simulink library "CRYP_PF_MASTER"  (Simulink 8.5)
settings: Solver=ode45  StartTime=0.0  StopTime=10.0  RelTol=1e-3
libraries: cdsEpicsOut x53, cdsFilt x16, cdsTP x16, VIS_LIB x8, cdsFunctionCall x5, cdsFiltCtrl x4, cdsMuxMatrix x4, cdsEpicsIn x2, lockin x2, QPD x2, cdsRms x2, FOUROSEM_COILOUTF_MASTER x1
(part 1 of 3)
settings Model: Creator=controls  LastModifiedBy=controls

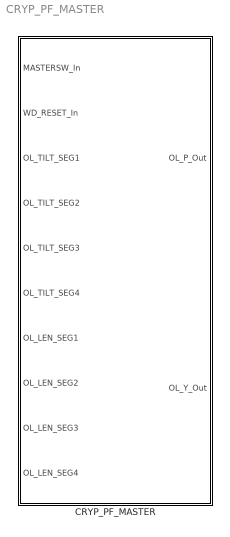
== system CRYP_PF_MASTER ==
  CRYP_PF_MASTER : Subsystem

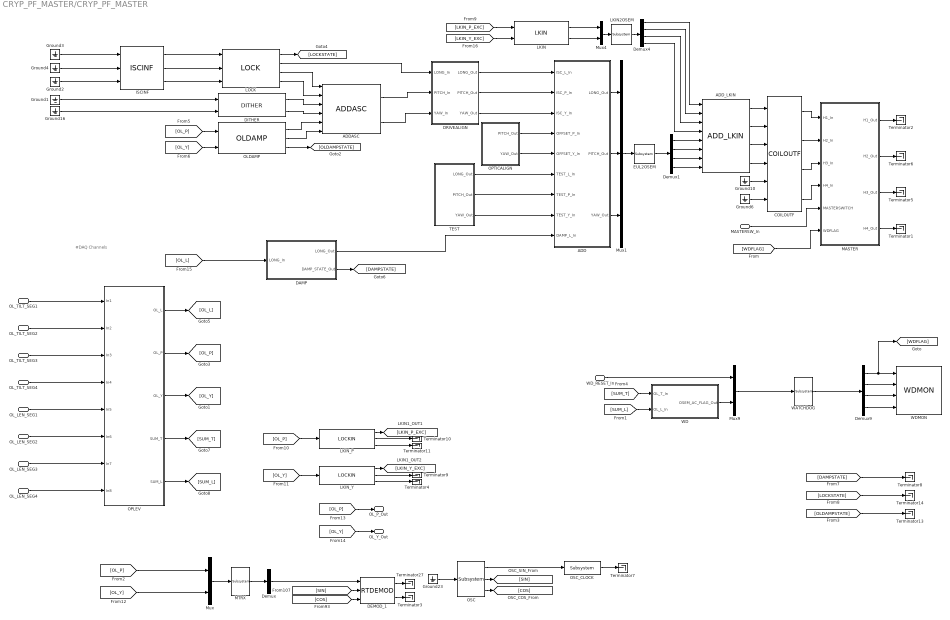
== system CRYP_PF_MASTER/CRYP_PF_MASTER ==
  note: #DAQ Channels
  MASTERSW_In : Inport
  WD_RESET_In : Inport  Port=2
  OL_TILT_SEG1 : Inport  Port=3
  OL_TILT_SEG2 : Inport  Port=4
  OL_TILT_SEG3 : Inport  Port=5
  OL_TILT_SEG4 : Inport  Port=6
  OL_LEN_SEG1 : Inport  Port=7
  OL_LEN_SEG2 : Inport  Port=8
  OL_LEN_SEG3 : Inport  Port=9
  OL_LEN_SEG4 : Inport  Port=10
  ADD : Subsystem
  ADDASC : VIS_LIB/ADDASC
  ADD_LKIN : VIS_LIB/ADD_LKIN
  COILOUTF : FOUROSEM_COILOUTF_MASTER/COILOUTF
  DAMP : Subsystem
  DEMOD_1 : rtdemod/RTDEMOD  Tag=top_names
  DITHER : VIS_LIB/DITHER
  DRIVEALIGN : Subsystem
  Demux : Demux  Outputs=1
  Demux1 : Demux
  Demux4 : Demux
  Demux9 : Demux
  EUL2OSEM : cdsMuxMatrix/Subsystem  Tag=cdsMuxMatrix  Description=Any size matrix. Inputs and outputs must be connected using Mux and Demux parts.
      settings: AttributesFormatString=%<Tag>
  Ground{1..4,6,10,16,23} (8 alike) : Ground
  ISCINF : VIS_LIB/ISCINF
  LKIN : VIS_LIB/LKIN
  LKIN2OSEM : cdsMuxMatrix/Subsystem  Tag=cdsMuxMatrix  Description=Any size matrix. Inputs and outputs must be connected using Mux and Demux parts.
      settings: AttributesFormatString=%<Tag>
  LKIN_P : lockin/LOCKIN  Description=ADL=LOCKIN.adl
      settings: AttributesFormatString=%<Tag>
  LKIN_Y : lockin/LOCKIN  Description=ADL=LOCKIN.adl
      settings: AttributesFormatString=%<Tag>
  LOCK : VIS_LIB/LOCK
  MASTER : Subsystem  AncestorBlock=VIS_LIB/MASTER
  MTRX : cdsMuxMatrix/Subsystem  Tag=cdsMuxMatrix  Description=Any size matrix. Inputs and outputs must be connected using Mux and Demux parts.
      settings: AttributesFormatString=%<Tag>
  Mux : Mux  Inputs=2
  Mux1 : Mux  Inputs=3
  Mux4 : Mux  Inputs=2
  Mux9 : Mux  Inputs=2
  OLDAMP : VIS_LIB/OLDAMP
  OPLEV : Subsystem
  OPTICALIGN : Subsystem
  OSC : cdsOsc/Subsystem  Tag=cdsOsc  Description=Oscillator
      settings: AttributesFormatString=%<Tag>
  OSC_CLOCK : cdsEpicsOut/Subsystem  Tag=cdsEpicsOutput  Description=|
      | Purpose:                                          
      | Output a FE signal to an EPICS channel.           
      |                                                   
      | Operation:                                        
      | Takes input value and passes it to EPICS record.  
      |                                                   
      | Usage:                                            
      | Name the part with the desired EPICS rrecord name.
      settings: AttributesFormatString=%<Tag>
  TEST : Subsystem
  Terminator{1..11,13..14,27} (14 alike) : Terminator
  WATCHDOG : cdsFunctionCall/Subsystem  Tag=cdsFunctionCall  Description=inline OSEMWATCHDOG /opt/rtcds/userapps/release/vis/common/src/WATCHDOG.c
      settings: AttributesFormatString=%<Tag>\n%<Description>
  WD : Subsystem
  WDMON : VIS_LIB/WDMON
  OL_P_Out : Outport
  OL_Y_Out : Outport  Port=2
  wires:
  [SUM_L] -> WD/2(OL_L_In)
  [SUM_T] -> WD/1(OL_T_In)
  DAMP/1(LONG_Out) -> ADD/9(DAMP_L_In)
  DAMP/2(DAMP_STATE_Out) -> [DAMPSTATE]
  [OL_L] -> DAMP/1(LONG_In)
  OPTICALIGN/2(YAW_Out) -> ADD/5(OFFSET_Y_In)
  OPTICALIGN/1(PITCH_Out) -> ADD/4(OFFSET_P_In)
  LOCK/3 -> ADDASC/1
  TEST/3(YAW_Out) -> ADD/8(TEST_Y_In)
  TEST/2(PITCH_Out) -> ADD/7(TEST_P_In)
  TEST/1(LONG_Out) -> ADD/6(TEST_L_In)
  Ground10/1 -> COILOUTF/5
  Ground6/1 -> COILOUTF/6
  WD_RESET_In/1 -> Mux9/1
  COILOUTF/4 -> MASTER/4(H4_In)
  COILOUTF/3 -> MASTER/3(H3_In)
  COILOUTF/2 -> MASTER/2(H2_In)
  COILOUTF/1 -> MASTER/1(H1_In)
  [WDFLAG] -> MASTER/6(WDFLAG)
  Mux9/1 -> WATCHDOG/1
  WATCHDOG/1 -> Demux9/1
  Demux9/4 -> WDMON/4
  Demux9/3 -> WDMON/3
  Demux9/2 -> WDMON/2
  Demux9/1 -> WDMON/1, [WDFLAG]
  EUL2OSEM/1 -> Demux1/1
  Mux1/1 -> EUL2OSEM/1
  Ground1/1 -> DITHER/1
  Ground16/1 -> DITHER/2
  [OL_P] -> OLDAMP/1
  [OL_Y] -> OLDAMP/2
  LOCK/4 -> ADDASC/2
  DITHER/1 -> ADDASC/3
  DITHER/2 -> ADDASC/4
  OLDAMP/1 -> ADDASC/5
  OLDAMP/2 -> ADDASC/6
  ADD/3(YAW_Out) -> Mux1/3
  ADD/2(PITCH_Out) -> Mux1/2
  ADD/1(LONG_Out) -> Mux1/1
  LOCK/2 -> DRIVEALIGN/1(LONG_In)
  ADDASC/1 -> DRIVEALIGN/2(PITCH_In)
  ADDASC/2 -> DRIVEALIGN/3(YAW_In)
  DRIVEALIGN/1(LONG_Out) -> ADD/1(ISC_L_In)
  DRIVEALIGN/2(PITCH_Out) -> ADD/2(ISC_P_In)
  DRIVEALIGN/3(YAW_Out) -> ADD/3(ISC_Y_In)
  OLDAMP/3 -> [OLDAMPSTATE]
  MASTER/1(H1_Out) -> Terminator2/1
  MASTER/2(H2_Out) -> Terminator6/1
  MASTER/3(H3_Out) -> Terminator5/1
  MASTER/4(H4_Out) -> Terminator1/1
  Mux4/1 -> LKIN2OSEM/1
  LKIN2OSEM/1 -> Demux4/1
  Demux4/1 -> ADD_LKIN/1
  LKIN/1 -> Mux4/1
  LKIN/2 -> Mux4/2
  Demux4/2 -> ADD_LKIN/2
  Demux4/3 -> ADD_LKIN/3
  Demux4/4 -> ADD_LKIN/4
  Demux1/1 -> ADD_LKIN/5
  Demux1/2 -> ADD_LKIN/6
  Demux1/3 -> ADD_LKIN/7
  Demux1/4 -> ADD_LKIN/8
  ADD_LKIN/1 -> COILOUTF/1
  ADD_LKIN/2 -> COILOUTF/2
  ADD_LKIN/3 -> COILOUTF/3
  ADD_LKIN/4 -> COILOUTF/4
  MASTERSW_In/1 -> MASTER/5(MASTERSWITCH)
  [DAMPSTATE] -> Terminator8/1
  [LOCKSTATE] -> Terminator14/1
  [OLDAMPSTATE] -> Terminator13/1
  LOCK/1 -> [LOCKSTATE]
  [LKIN_P_EXC] -> LKIN/1
  [LKIN_Y_EXC] -> LKIN/2
  WD/1(OSEM_AC_FLAG_Out) -> Mux9/2
  Ground2/1 -> ISCINF/3
  Ground3/1 -> ISCINF/1
  Ground4/1 -> ISCINF/2
  ISCINF/1 -> LOCK/1
  ISCINF/2 -> LOCK/2
  ISCINF/3 -> LOCK/3
  Mux/1 -> MTRX/1
  MTRX/1 -> Demux/1
  Demux/1 -> DEMOD_1/1
  [SIN] -> DEMOD_1/2
  [COS] -> DEMOD_1/3
  DEMOD_1/1 -> Terminator27/1
  DEMOD_1/2 -> Terminator3/1
  Ground23/1 -> OSC/1
  OSC/1 -> OSC_CLOCK/1
  OSC_CLOCK/1 -> Terminator7/1
  OSC/2 -> [SIN]
  OSC/3 -> [COS]
  [OL_P] -> Mux/1
  [OL_Y] -> Mux/2
  [OL_P] -> LKIN_P/1
  LKIN_P/2 -> Terminator10/1
  LKIN_P/3 -> Terminator11/1
  LKIN_P/1 -> [LKIN_P_EXC]
  LKIN_Y/1 -> [LKIN_Y_EXC]
  [OL_Y] -> LKIN_Y/1
  LKIN_Y/2 -> Terminator9/1
  LKIN_Y/3 -> Terminator4/1
  [OL_P] -> OL_P_Out/1
  [OL_Y] -> OL_Y_Out/1
  OPLEV/5(SUM_L) -> [SUM_L]
  OPLEV/4(SUM_T) -> [SUM_T]
  OPLEV/3(OL_Y) -> [OL_Y]
  OPLEV/2(OL_P) -> [OL_P]
  OPLEV/1(OL_L) -> [OL_L]
  OL_TILT_SEG3/1 -> OPLEV/3(In3)
  OL_LEN_SEG4/1 -> OPLEV/8(In8)
  OL_LEN_SEG3/1 -> OPLEV/7(In7)
  OL_LEN_SEG2/1 -> OPLEV/6(In6)
  OL_LEN_SEG1/1 -> OPLEV/5(In5)
  OL_TILT_SEG4/1 -> OPLEV/4(In4)
  OL_TILT_SEG2/1 -> OPLEV/2(In2)
  OL_TILT_SEG1/1 -> OPLEV/1(In1)

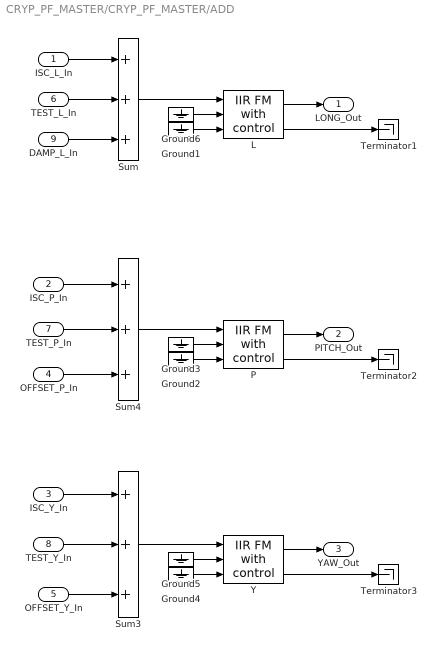
== system CRYP_PF_MASTER/CRYP_PF_MASTER/ADD ==
  ISC_L_In : Inport
  ISC_P_In : Inport  Port=2
  ISC_Y_In : Inport  Port=3
  OFFSET_P_In : Inport  Port=4
  OFFSET_Y_In : Inport  Port=5
  TEST_L_In : Inport  Port=6
  TEST_P_In : Inport  Port=7
  TEST_Y_In : Inport  Port=8
  DAMP_L_In : Inport  Port=9
  Ground{1..6} (6 alike) : Ground
  L : cdsFiltCtrl/IIR FM with control  Tag=cdsFiltCtrl  Description=|
      | cdsFiltCntrl is the standard IIR filter module (exactly the same as cdsFilt) but with added control data output 'Ctrl'. Filter module digital signal output appears on the first output, which is called 'Val'. 'Ctrl' output has a bit pattern encoding the state of filter's on/off switches (FM1 through FM10). The bit values are:
      |                                                                                                                                                                                                                                                                                                                                       
      | module 	hex	dec                                                                                                                                                                                                                                                                                                                       
      | -----------------------                                                                                                                                                                                                                                                                                                               
      | FM1	0x20                    32                                                                                                                                                                                                                                                                                                        
      | FM2	0x80                     128                                                                                                                                                                                                                                                                                                      
      | FM3	0x200                   512                                                                                                                                                                                                                                                                                                       
      | FM4	0x800                   2048                                                                                                                                                                                                                                                                                                      
      | FM5	0x2000                 8192                                                                                                                                                                                                                                                                                                       
      | FM6	0x8000                 32768                                                                                                                                                                                                                                                                                                      
      | FM7	0x20000                131072                                                                                                                                                                                                                                                                                                     
      | FM8	0x80000                 524288                                                                                                                                                                                                                                                                                                    
      | FM9	0x200000               2097152                                                                                                                                                                                                                                                                                                    
      | FM10	0x800000               8388608                                                                                                                                                                                                                                                                                                   
      |                                                                                                                                                                                                                                                                                                                                       
      | This bit data can be used to drive some other switches or it can be output using a binary I/O module.
      settings: AttributesFormatString=%<Tag>
  P : cdsFiltCtrl/IIR FM with control  Tag=cdsFiltCtrl  Description=|
      | cdsFiltCntrl is the standard IIR filter module (exactly the same as cdsFilt) but with added control data output 'Ctrl'. Filter module digital signal output appears on the first output, which is called 'Val'. 'Ctrl' output has a bit pattern encoding the state of filter's on/off switches (FM1 through FM10). The bit values are:
      |                                                                                                                                                                                                                                                                                                                                       
      | module 	hex	dec                                                                                                                                                                                                                                                                                                                       
      | -----------------------                                                                                                                                                                                                                                                                                                               
      | FM1	0x20                    32                                                                                                                                                                                                                                                                                                        
      | FM2	0x80                     128                                                                                                                                                                                                                                                                                                      
      | FM3	0x200                   512                                                                                                                                                                                                                                                                                                       
      | FM4	0x800                   2048                                                                                                                                                                                                                                                                                                      
      | FM5	0x2000                 8192                                                                                                                                                                                                                                                                                                       
      | FM6	0x8000                 32768                                                                                                                                                                                                                                                                                                      
      | FM7	0x20000                131072                                                                                                                                                                                                                                                                                                     
      | FM8	0x80000                 524288                                                                                                                                                                                                                                                                                                    
      | FM9	0x200000               2097152                                                                                                                                                                                                                                                                                                    
      | FM10	0x800000               8388608                                                                                                                                                                                                                                                                                                   
      |                                                                                                                                                                                                                                                                                                                                       
      | This bit data can be used to drive some other switches or it can be output using a binary I/O module.
      settings: AttributesFormatString=%<Tag>
  Sum : Sum  Inputs=+++
  Sum3 : Sum  Inputs=+++
  Sum4 : Sum  Inputs=+++
  Terminator1 : Terminator
  Terminator2 : Terminator
  Terminator3 : Terminator
  Y : cdsFiltCtrl/IIR FM with control  Tag=cdsFiltCtrl  Description=|
      | cdsFiltCntrl is the standard IIR filter module (exactly the same as cdsFilt) but with added control data output 'Ctrl'. Filter module digital signal output appears on the first output, which is called 'Val'. 'Ctrl' output has a bit pattern encoding the state of filter's on/off switches (FM1 through FM10). The bit values are:
      |                                                                                                                                                                                                                                                                                                                                       
      | module 	hex	dec                                                                                                                                                                                                                                                                                                                       
      | -----------------------                                                                                                                                                                                                                                                                                                               
      | FM1	0x20                    32                                                                                                                                                                                                                                                                                                        
      | FM2	0x80                     128                                                                                                                                                                                                                                                                                                      
      | FM3	0x200                   512                                                                                                                                                                                                                                                                                                       
      | FM4	0x800                   2048                                                                                                                                                                                                                                                                                                      
      | FM5	0x2000                 8192                                                                                                                                                                                                                                                                                                       
      | FM6	0x8000                 32768                                                                                                                                                                                                                                                                                                      
      | FM7	0x20000                131072                                                                                                                                                                                                                                                                                                     
      | FM8	0x80000                 524288                                                                                                                                                                                                                                                                                                    
      | FM9	0x200000               2097152                                                                                                                                                                                                                                                                                                    
      | FM10	0x800000               8388608                                                                                                                                                                                                                                                                                                   
      |                                                                                                                                                                                                                                                                                                                                       
      | This bit data can be used to drive some other switches or it can be output using a binary I/O module.
      settings: AttributesFormatString=%<Tag>
  LONG_Out : Outport
  PITCH_Out : Outport  Port=2
  YAW_Out : Outport  Port=3
  wires:
  DAMP_L_In/1 -> Sum/3
  OFFSET_P_In/1 -> Sum4/3
  OFFSET_Y_In/1 -> Sum3/3
  ISC_L_In/1 -> Sum/1
  TEST_L_In/1 -> Sum/2
  ISC_Y_In/1 -> Sum3/1
  TEST_Y_In/1 -> Sum3/2
  TEST_P_In/1 -> Sum4/2
  ISC_P_In/1 -> Sum4/1
  Sum/1 -> L/1
  Ground1/1 -> L/3
  Ground6/1 -> L/2
  L/1 -> LONG_Out/1
  Sum4/1 -> P/1
  Ground2/1 -> P/3
  Ground3/1 -> P/2
  P/1 -> PITCH_Out/1
  Sum3/1 -> Y/1
  Ground4/1 -> Y/3
  Ground5/1 -> Y/2
  Y/1 -> YAW_Out/1
  L/2 -> Terminator1/1
  P/2 -> Terminator2/1
  Y/2 -> Terminator3/1

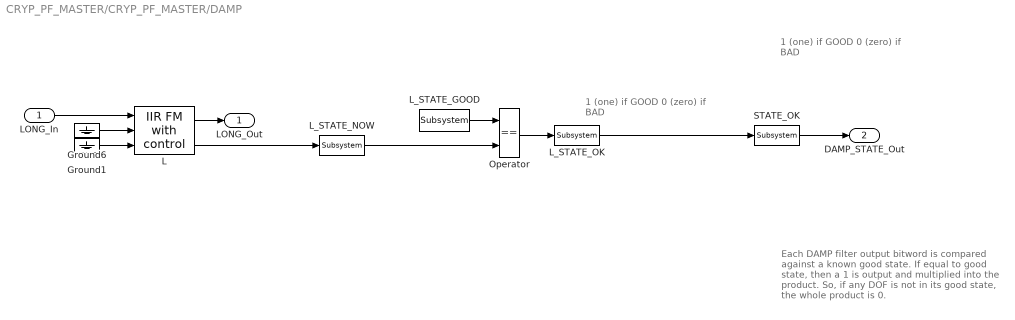
== system CRYP_PF_MASTER/CRYP_PF_MASTER/DAMP ==
  note: Each DAMP filter output bitword is
      | compared against a known good state.
      | If equal to good state, then a 1 is output
      | and multiplied into the product. So, if any DOF
      | is not in its good state, the whole product is 0.
  note: 1 (one) if GOOD
      | 0 (zero) if BAD
  note: 1 (one) if GOOD
      | 0 (zero) if BAD
  LONG_In : Inport
  Ground1 : Ground
  Ground6 : Ground
  L : cdsFiltCtrl/IIR FM with control  Tag=cdsFiltCtrl  Description=|
      | cdsFiltCntrl is the standard IIR filter module (exactly the same as cdsFilt) but with added control data output 'Ctrl'. Filter module digital signal output appears on the first output, which is called 'Val'. 'Ctrl' output has a bit pattern encoding the state of filter's on/off switches (FM1 through FM10). The bit values are:
      |                                                                                                                                                                                                                                                                                                                                       
      | module 	hex	dec                                                                                                                                                                                                                                                                                                                       
      | -----------------------                                                                                                                                                                                                                                                                                                               
      | FM1	0x20                    32                                                                                                                                                                                                                                                                                                        
      | FM2	0x80                     128                                                                                                                                                                                                                                                                                                      
      | FM3	0x200                   512                                                                                                                                                                                                                                                                                                       
      | FM4	0x800                   2048                                                                                                                                                                                                                                                                                                      
      | FM5	0x2000                 8192                                                                                                                                                                                                                                                                                                       
      | FM6	0x8000                 32768                                                                                                                                                                                                                                                                                                      
      | FM7	0x20000                131072                                                                                                                                                                                                                                                                                                     
      | FM8	0x80000                 524288                                                                                                                                                                                                                                                                                                    
      | FM9	0x200000               2097152                                                                                                                                                                                                                                                                                                    
      | FM10	0x800000               8388608                                                                                                                                                                                                                                                                                                   
      |                                                                                                                                                                                                                                                                                                                                       
      | This bit data can be used to drive some other switches or it can be output using a binary I/O module.
      settings: AttributesFormatString=%<Tag>
  L_STATE_GOOD : cdsEpicsIn/Subsystem  Tag=cdsEpicsIn  Description=|
      | Purpose:                                                                              
      | Create an EPICS input channel connection to the FE realtime controls.                 
      |                                                                                       
      | Operation:                                                                            
      | Outputs value from an EPICS ai record. Value is floating point with a precision of 3..
      |                                                                                       
      | Usage:                                                                                
      | Name the part with the desired EPICS channel name.
      settings: AttributesFormatString=%<Tag>
  L_STATE_NOW : cdsEpicsOut/Subsystem  Tag=cdsEpicsOutput  Description=|
      | Purpose:                                          
      | Output a FE signal to an EPICS channel.           
      |                                                   
      | Operation:                                        
      | Takes input value and passes it to EPICS record.  
      |                                                   
      | Usage:                                            
      | Name the part with the desired EPICS rrecord name.
      settings: AttributesFormatString=%<Tag>
  L_STATE_OK : cdsEpicsOut/Subsystem  Tag=cdsEpicsOutput  Description=|
      | Purpose:                                          
      | Output a FE signal to an EPICS channel.           
      |                                                   
      | Operation:                                        
      | Takes input value and passes it to EPICS record.  
      |                                                   
      | Usage:                                            
      | Name the part with the desired EPICS rrecord name.
      settings: AttributesFormatString=%<Tag>
  Operator : RelationalOperator  Operator===  OutDataTypeStr=boolean
  STATE_OK : cdsEpicsOut/Subsystem  Tag=cdsEpicsOutput  Description=|
      | Purpose:                                          
      | Output a FE signal to an EPICS channel.           
      |                                                   
      | Operation:                                        
      | Takes input value and passes it to EPICS record.  
      |                                                   
      | Usage:                                            
      | Name the part with the desired EPICS rrecord name.
      settings: AttributesFormatString=%<Tag>
  LONG_Out : Outport
  DAMP_STATE_Out : Outport  Port=2
  wires:
  Ground1/1 -> L/3
  Ground6/1 -> L/2
  LONG_In/1 -> L/1
  L/1 -> LONG_Out/1
  L_STATE_GOOD/1 -> Operator/1
  L/2 -> L_STATE_NOW/1
  L_STATE_OK/1 -> STATE_OK/1
  Operator/1 -> L_STATE_OK/1
  L_STATE_NOW/1 -> Operator/2
  STATE_OK/1 -> DAMP_STATE_Out/1
